simulink model "untitled"  (R2021b)
settings: Solver=VariableStepAuto  StartTime=0.0  StopTime=10.0  RelTol=1e-3
undefined symbols (not defined in the file): p
settings Model: Creator=nan  LastModifiedBy=nan

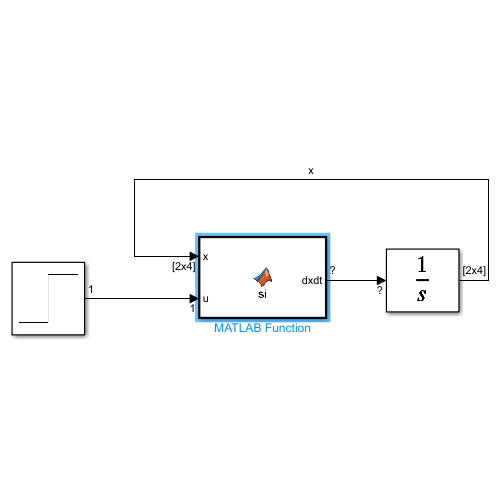
[thumbnail: Simulink's stored preview of the top-level diagram]
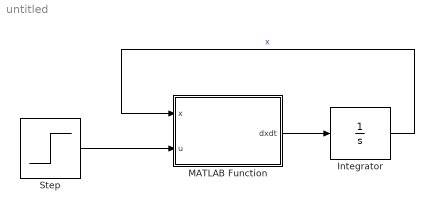
== system untitled ==
  Integrator : Integrator  InitialCondition=[1-p;p]
  MATLAB Function : MATLAB Function  TreatAsAtomicUnit=on
  Step : Step  Time=5  After=0.8  SampleTime=0
  wires:
  MATLAB Function/1(dxdt) -> Integrator/1
  Integrator/1 -> MATLAB Function/1(x)  "x"
  Step/1 -> MATLAB Function/2(u)

== matlab function untitled/MATLAB Function ==
  data: x input; u input; dxdt output
function dxdt = si(x, u)
beta = 0.8;
gamma = 0.1;
delta = 0.02;
dxdt = [-beta * (1 - u) * x(1) * x(2);
    beta * (1 - u) * x(1) * x(2) - gamma * x(2) - delta * x(2)];
end
